simulink subsystem "HallSensor"  (R2023a)
settings: Solver=VariableStepAuto  StartTime=0.0  StopTime=10.0  RelTol=1e-3
settings Model: Creator=lehas  LastModifiedBy=lehas

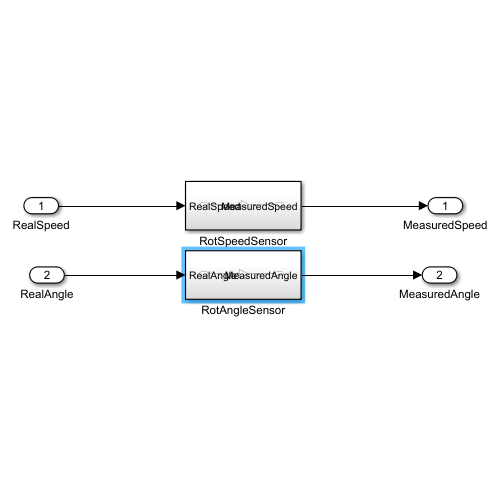
[thumbnail: Simulink's stored preview of the top-level diagram]
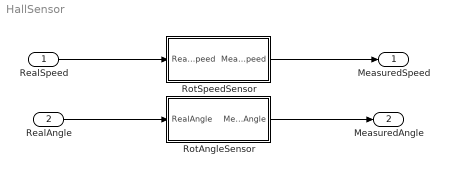
== system HallSensor ==
  RealSpeed : Inport
  RealAngle : Inport  Port=2
  RotAngleSensor : Subsystem
  RotSpeedSensor : Subsystem
  MeasuredSpeed : Outport
  MeasuredAngle : Outport  Port=2
  wires:
  RealSpeed/1 -> RotSpeedSensor/1(RealSpeed)
  RotSpeedSensor/1(MeasuredSpeed) -> MeasuredSpeed/1
  RealAngle/1 -> RotAngleSensor/1(RealAngle)
  RotAngleSensor/1(MeasuredAngle) -> MeasuredAngle/1

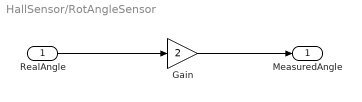
== system HallSensor/RotAngleSensor ==
  RealAngle : Inport
  Gain : Gain  Gain=2
  MeasuredAngle : Outport
  wires:
  RealAngle/1 -> Gain/1
  Gain/1 -> MeasuredAngle/1

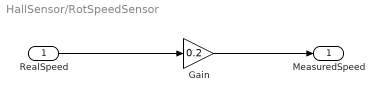
== system HallSensor/RotSpeedSensor ==
  RealSpeed : Inport
  Gain : Gain  Gain=0.2
  MeasuredSpeed : Outport
  wires:
  RealSpeed/1 -> Gain/1
  Gain/1 -> MeasuredSpeed/1
